simulink library "mnNb_Lib"  (R2016a)
settings: Solver=ode45  StartTime=0.0  StopTime=10.0  RelTol=1e-3
undefined symbols (not defined in the file): AA_AI, Chan, CMS_Elec, CMS_SW, FB, FB_SW, FB_SW_TTFSS, TTFSS_Elec, TTFSS_Gain
libraries: cstblocks x37, NbLibrary x33, mnNb_Lib x17
settings Model: Creator=Masayuki  LastModifiedBy=Masayuki
settings DataIOCC: LimitDataPoints=on
settings DebuggingCC: AllowSymbolicDim=off

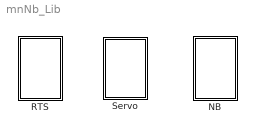
== system mnNb_Lib ==
  NB : Subsystem
  RTS : Subsystem
  Servo : Subsystem

== system mnNb_Lib/NB ==
  "NBpoint " : Subsystem  mask{DOF=''}
  NBsink : Subsystem  mask{DOF='', asd=sp}
      mask prompts: asd "Amplitude spectral density"
      mask TypeOptions asd: NbSink/asd | NbSink_CMS_CARM/asd | NbSink_CMS_IMC/asd | NbSink_FSSpath/asd | NbSink_IMCpath/asd | NbSink_TTFSS/asd | NbSink_act_AOM/asd | NbSink_act_EOM/asd | NbSink_act_IMCsus/asd | NbSink_act_PZT/asd | NbSink_act_TEMP/asd | NbSink_laser/asd | NbSink_motion_RC/asd | NbSink_seismic_CARM/asd | NbSink_seismic_IMC/asd | NbSink_shot_CARM/asd | NbSink_shot_IMC/asd | NbSink_shot_RC/asd | NbSink_sensor_IMC/asd | NbSink_sensor_RC/asd
  NoiseSource : Subsystem  mask{DOF='', group='', unit='', asd=sp}
      mask prompts: DOF "Noise name"; asd "Amplitude spectral density"
      mask TypeOptions asd: Nbsource/asd

== system mnNb_Lib/RTS ==
  ADC : Subsystem
  DAC : Subsystem
  FB_module : Subsystem
  mn Filter Bank : Subsystem  mask{Chan=Chan, FB=FB, FB_SW=FB_SW}
      mask prompts: Chan "Channel Name"; FB "FB filters container"; FB_SW "FB switch container"
      mask TypeOptions Chan: FB1/Chan | FB10/Chan | FB2/Chan | FB3/Chan | FB4/Chan | FB5/Chan | FB6/Chan | FB7/Chan | FB8/Chan | FB9/Chan
      mask TypeOptions FB: FB1/FB | FB10/FB | FB2/FB | FB3/FB | FB4/FB | FB5/FB | FB6/FB | FB7/FB | FB8/FB | FB9/FB
      mask TypeOptions FB_SW: FB1/FB_SW | FB10/FB_SW | FB2/FB_SW | FB3/FB_SW | FB4/FB_SW | FB5/FB_SW | FB6/FB_SW | FB7/FB_SW | FB8/FB_SW | FB9/FB_SW | Gain/FB_SW

== system mnNb_Lib/Servo ==
  Common Mode Servo : Subsystem  mask{CMS_Elec=CMS_Elec, CMS_SW=CMS_SW}
      mask prompts: CMS_Elec "transfer function containers"; CMS_SW "switch containers"
  TTFSS : Subsystem  mask{Elec=TTFSS_Elec, TTFSS_Gain=TTFSS_Gain, FB=FB, Chan='K1:PSL-TTFSS_TEMP_FILTER', RTS=FB_SW_TTFSS}
      mask prompts: Elec "Transfer function container"; TTFSS_Gain "Gain container"; FB "FB filters container"; Chan "Temperature control channel Name"; RTS "temperature control filters container"
      mask TypeOptions FB: TEMP Filter/FB
      mask TypeOptions Chan: TEMP Filter/Chan
      mask TypeOptions RTS: TEMP Filter/FB_SW

== system mnNb_Lib/NB/NBpoint  ==
  In1 : Inport
  NbCal : NbLibrary/NbNoiseCal  Tag=NbNoiseCal  dof=DOF  unit='control signal [V/rtHz]'
      settings: AttributesFormatString=%<Tag>
  NbSink : NbLibrary/NbNoiseSink  Tag=NbNoiseSink  dof=DOF  asd=sp  chan=''
      settings: AttributesFormatString=%<Tag>
  Sum12 : Sum  Inputs=|++
  Terminator : Terminator
  wires:
  Sum12/1 -> NbSink/1
  NbSink/1 -> Terminator/1
  In1/1 -> Sum12/1
  NbCal/1 -> Sum12/2

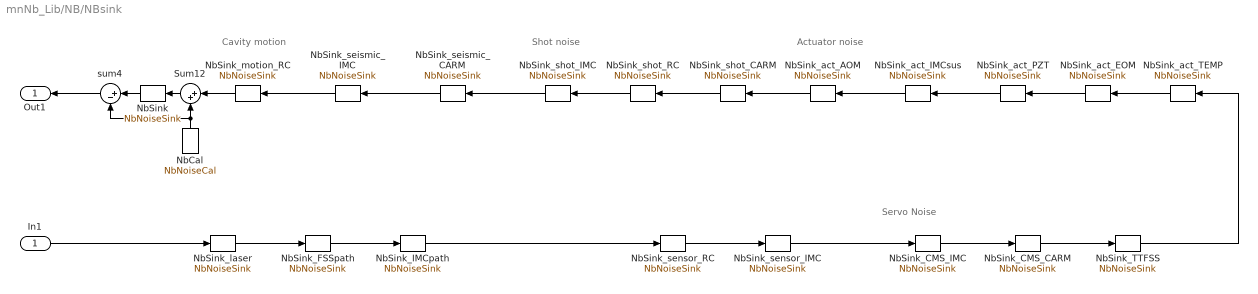
== system mnNb_Lib/NB/NBsink ==
  note: Servo Noise
  note: Actuator noise
  note: Shot noise
  note: Cavity motion
  In1 : Inport
  NbCal : NbLibrary/NbNoiseCal  Tag=NbNoiseCal  dof=DOF  unit='voltage [V/rHz]'
      settings: AttributesFormatString=%<Tag>
  NbSink : NbLibrary/NbNoiseSink  Tag=NbNoiseSink  dof=DOF  asd=sp  chan=''
      settings: AttributesFormatString=%<Tag>
  NbSink_CMS_CARM : NbLibrary/NbNoiseSink  Tag=NbNoiseSink  dof=[DOF '_CMS_CARM']  asd=sp  chan=''
      settings: AttributesFormatString=%<Tag>
  NbSink_CMS_IMC : NbLibrary/NbNoiseSink  Tag=NbNoiseSink  dof=[DOF '_CMS_IMC']  asd=sp  chan=''
      settings: AttributesFormatString=%<Tag>
  NbSink_FSSpath : NbLibrary/NbNoiseSink  Tag=NbNoiseSink  dof=[DOF '_freq_FSSpath']  asd=sp  chan=''
      settings: AttributesFormatString=%<Tag>
  NbSink_IMCpath : NbLibrary/NbNoiseSink  Tag=NbNoiseSink  dof=[DOF '_freq_IMCpath']  asd=sp  chan=''
      settings: AttributesFormatString=%<Tag>
  NbSink_TTFSS : NbLibrary/NbNoiseSink  Tag=NbNoiseSink  dof=[DOF '_TTFSS']  asd=sp  chan=''
      settings: AttributesFormatString=%<Tag>
  NbSink_act_AOM : NbLibrary/NbNoiseSink  Tag=NbNoiseSink  dof=[DOF '_act_AOM']  asd=sp  chan=''
      settings: AttributesFormatString=%<Tag>
  NbSink_act_EOM : NbLibrary/NbNoiseSink  Tag=NbNoiseSink  dof=[DOF '_act_EOM']  asd=sp  chan=''
      settings: AttributesFormatString=%<Tag>
  NbSink_act_IMCsus : NbLibrary/NbNoiseSink  Tag=NbNoiseSink  dof=[DOF '_act_IMCsus']  asd=sp  chan=''
      settings: AttributesFormatString=%<Tag>
  NbSink_act_PZT : NbLibrary/NbNoiseSink  Tag=NbNoiseSink  dof=[DOF '_act_PZT']  asd=sp  chan=''
      settings: AttributesFormatString=%<Tag>
  NbSink_act_TEMP : NbLibrary/NbNoiseSink  Tag=NbNoiseSink  dof=[DOF '_act_TEMP']  asd=sp  chan=''
      settings: AttributesFormatString=%<Tag>
  NbSink_laser : NbLibrary/NbNoiseSink  Tag=NbNoiseSink  dof=[DOF '_NPRO']  asd=sp  chan=''
      settings: AttributesFormatString=%<Tag>
  NbSink_motion_RC : NbLibrary/NbNoiseSink  Tag=NbNoiseSink  dof=[DOF '_motion_RefCav']  asd=sp  chan=''
      settings: AttributesFormatString=%<Tag>
  NbSink_seismic_CARM : NbLibrary/NbNoiseSink  Tag=NbNoiseSink  dof=[DOF '_seismic_CARM']  asd=sp  chan=''
      settings: AttributesFormatString=%<Tag>
  NbSink_seismic_IMC : NbLibrary/NbNoiseSink  Tag=NbNoiseSink  dof=[DOF '_seismic_IMC']  asd=sp  chan=''
      settings: AttributesFormatString=%<Tag>
  NbSink_sensor_IMC : NbLibrary/NbNoiseSink  Tag=NbNoiseSink  dof=[DOF '_sensor_IMC']  asd=sp  chan=''
      settings: AttributesFormatString=%<Tag>
  NbSink_sensor_RC : NbLibrary/NbNoiseSink  Tag=NbNoiseSink  dof=[DOF '_sensor_RefCav']  asd=sp  chan=''
      settings: AttributesFormatString=%<Tag>
  NbSink_shot_CARM : NbLibrary/NbNoiseSink  Tag=NbNoiseSink  dof=[DOF '_shot_CARM']  asd=sp  chan=''
      settings: AttributesFormatString=%<Tag>
  NbSink_shot_IMC : NbLibrary/NbNoiseSink  Tag=NbNoiseSink  dof=[DOF '_shot_IMC']  asd=sp  chan=''
      settings: AttributesFormatString=%<Tag>
  NbSink_shot_RC : NbLibrary/NbNoiseSink  Tag=NbNoiseSink  dof=[DOF '_shot_RefCav']  asd=sp  chan=''
      settings: AttributesFormatString=%<Tag>
  Sum12 : Sum  Inputs=|++
  sum4 : Sum  Inputs=|+-
  Out1 : Outport
  wires:
  Sum12/1 -> NbSink/1
  NbSink/1 -> sum4/1
  NbCal/1 -> sum4/2, Sum12/2
  sum4/1 -> Out1/1
  In1/1 -> NbSink_laser/1
  NbSink_motion_RC/1 -> Sum12/1
  NbSink_act_AOM/1 -> NbSink_shot_CARM/1
  NbSink_TTFSS/1 -> NbSink_act_TEMP/1
  NbSink_CMS_IMC/1 -> NbSink_CMS_CARM/1
  NbSink_shot_IMC/1 -> NbSink_seismic_CARM/1
  NbSink_shot_RC/1 -> NbSink_shot_IMC/1
  NbSink_seismic_IMC/1 -> NbSink_motion_RC/1
  NbSink_seismic_CARM/1 -> NbSink_seismic_IMC/1
  NbSink_shot_CARM/1 -> NbSink_shot_RC/1
  NbSink_act_IMCsus/1 -> NbSink_act_AOM/1
  NbSink_act_PZT/1 -> NbSink_act_IMCsus/1
  NbSink_act_EOM/1 -> NbSink_act_PZT/1
  NbSink_act_TEMP/1 -> NbSink_act_EOM/1
  NbSink_CMS_CARM/1 -> NbSink_TTFSS/1
  NbSink_laser/1 -> NbSink_FSSpath/1
  NbSink_FSSpath/1 -> NbSink_IMCpath/1
  NbSink_IMCpath/1 -> NbSink_sensor_RC/1
  NbSink_sensor_IMC/1 -> NbSink_CMS_IMC/1
  NbSink_sensor_RC/1 -> NbSink_sensor_IMC/1

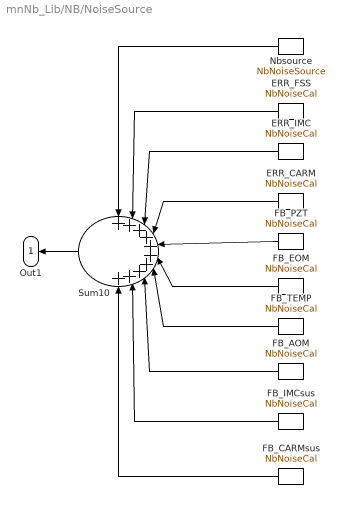
== system mnNb_Lib/NB/NoiseSource ==
  ERR_CARM : NbLibrary/NbNoiseCal  Tag=NbNoiseCal  dof=['ERR_CARM_' DOF]  unit=unit
      settings: AttributesFormatString=%<Tag>
  ERR_FSS : NbLibrary/NbNoiseCal  Tag=NbNoiseCal  dof=['ERR_FSS_' DOF]  unit=unit
      settings: AttributesFormatString=%<Tag>
  ERR_IMC : NbLibrary/NbNoiseCal  Tag=NbNoiseCal  dof=['ERR_IMC_' DOF]  unit=unit
      settings: AttributesFormatString=%<Tag>
  FB_AOM : NbLibrary/NbNoiseCal  Tag=NbNoiseCal  dof=['FB_AOM_' DOF]  unit=unit
      settings: AttributesFormatString=%<Tag>
  FB_CARMsus : NbLibrary/NbNoiseCal  Tag=NbNoiseCal  dof=['FB_CARMsus_' DOF]  unit=unit
      settings: AttributesFormatString=%<Tag>
  FB_EOM : NbLibrary/NbNoiseCal  Tag=NbNoiseCal  dof=['FB_EOM_' DOF]  unit=unit
      settings: AttributesFormatString=%<Tag>
  FB_IMCsus : NbLibrary/NbNoiseCal  Tag=NbNoiseCal  dof=['FB_IMCsus_' DOF]  unit=unit
      settings: AttributesFormatString=%<Tag>
  FB_PZT : NbLibrary/NbNoiseCal  Tag=NbNoiseCal  dof=['FB_PZT_' DOF]  unit=unit
      settings: AttributesFormatString=%<Tag>
  FB_TEMP : NbLibrary/NbNoiseCal  Tag=NbNoiseCal  dof=['FB_TEMP_' DOF]  unit=unit
      settings: AttributesFormatString=%<Tag>
  Nbsource : NbLibrary/NbNoiseSource  Tag=NbNoiseSource  asd=sp  chan=''  groupNest=1  group=group  subgroup=''  subsubgroup=''  subsubsubgroup=''
      settings: AttributesFormatString=%<Tag>
  Sum10 : Sum  Inputs=++++++++++
  Out1 : Outport
  wires:
  Nbsource/1 -> Sum10/1
  Sum10/1 -> Out1/1
  ERR_FSS/1 -> Sum10/2
  ERR_IMC/1 -> Sum10/3
  ERR_CARM/1 -> Sum10/4
  FB_PZT/1 -> Sum10/5
  FB_EOM/1 -> Sum10/6
  FB_TEMP/1 -> Sum10/7
  FB_AOM/1 -> Sum10/8
  FB_IMCsus/1 -> Sum10/9
  FB_CARMsus/1 -> Sum10/10

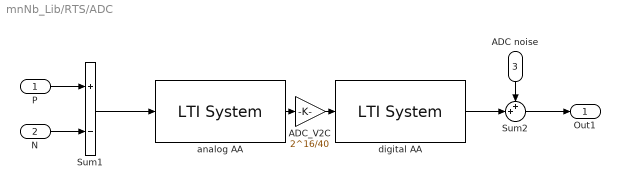
== system mnNb_Lib/RTS/ADC ==
  P : Inport
  N : Inport  Port=2
  ADC noise : Inport  Port=3
  ADC_V2C : Gain  Gain=2^16/40
  Sum1 : Sum  Inputs=+-
  Sum2 : Sum  Inputs=++|
  analog AA : cstblocks/LTI System  sys=AA_AI('Analog_AA')  IC=[]
  digital AA : cstblocks/LTI System  sys=AA_AI('Digital_AA')  IC=[]
  Out1 : Outport
  wires:
  analog AA/1 -> ADC_V2C/1
  ADC_V2C/1 -> digital AA/1
  P/1 -> Sum1/1
  N/1 -> Sum1/2
  digital AA/1 -> Sum2/2
  Sum2/1 -> Out1/1
  ADC noise/1 -> Sum2/1
  Sum1/1 -> analog AA/1

== system mnNb_Lib/RTS/DAC ==
  In1 : Inport
  DAC noise : Inport  Port=2
  DAC_C2V : Gain  Gain=20/2^16
  Sum2 : Sum  Inputs=++|
  analog AI : cstblocks/LTI System  sys=AA_AI('Analog_AI')  IC=[]
  digital AI : cstblocks/LTI System  sys=AA_AI('Digital_AI')  IC=[]
  n : Gain  Gain=-1
  P : Outport
  N : Outport  Port=2
  wires:
  In1/1 -> analog AI/1
  analog AI/1 -> DAC_C2V/1
  DAC_C2V/1 -> digital AI/1
  n/1 -> N/1
  DAC noise/1 -> Sum2/1
  digital AI/1 -> Sum2/2
  Sum2/1 -> P/1, n/1

== system mnNb_Lib/RTS/FB_module ==
  FB1 : Subsystem  mask{i=1, Chan=Chan, FB=FB, FB_SW=FB_SW}
      mask prompts: i "FB No"; Chan "Channel Name"; FB "FB filters container"; FB_SW "FB switch container"

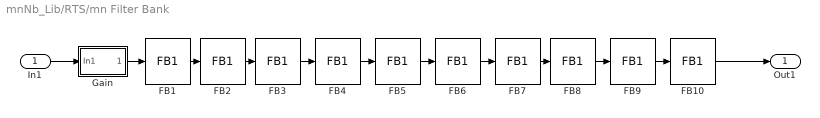
== system mnNb_Lib/RTS/mn Filter Bank ==
  In1 : Inport
  FB1 : mnNb_Lib/RTS/FB_module/FB1  i=1  Chan=Chan  FB=FB  FB_SW=FB_SW
  FB10 : mnNb_Lib/RTS/FB_module/FB1  i=10  Chan=Chan  FB=FB  FB_SW=FB_SW
  FB2 : mnNb_Lib/RTS/FB_module/FB1  i=2  Chan=Chan  FB=FB  FB_SW=FB_SW
  FB3 : mnNb_Lib/RTS/FB_module/FB1  i=3  Chan=Chan  FB=FB  FB_SW=FB_SW
  FB4 : mnNb_Lib/RTS/FB_module/FB1  i=4  Chan=Chan  FB=FB  FB_SW=FB_SW
  FB5 : mnNb_Lib/RTS/FB_module/FB1  i=5  Chan=Chan  FB=FB  FB_SW=FB_SW
  FB6 : mnNb_Lib/RTS/FB_module/FB1  i=6  Chan=Chan  FB=FB  FB_SW=FB_SW
  FB7 : mnNb_Lib/RTS/FB_module/FB1  i=7  Chan=Chan  FB=FB  FB_SW=FB_SW
  FB8 : mnNb_Lib/RTS/FB_module/FB1  i=8  Chan=Chan  FB=FB  FB_SW=FB_SW
  FB9 : mnNb_Lib/RTS/FB_module/FB1  i=9  Chan=Chan  FB=FB  FB_SW=FB_SW
  Gain : Subsystem  mask{FB_SW=FB_SW}
      mask prompts: FB_SW "gain container"
  Out1 : Outport
  wires:
  FB10/1 -> Out1/1
  FB1/1 -> FB2/1
  FB2/1 -> FB3/1
  FB3/1 -> FB4/1
  FB4/1 -> FB5/1
  FB5/1 -> FB6/1
  FB6/1 -> FB7/1
  FB7/1 -> FB8/1
  FB8/1 -> FB9/1
  FB9/1 -> FB10/1
  In1/1 -> Gain/1(In1)
  Gain/1(Out1) -> FB1/1

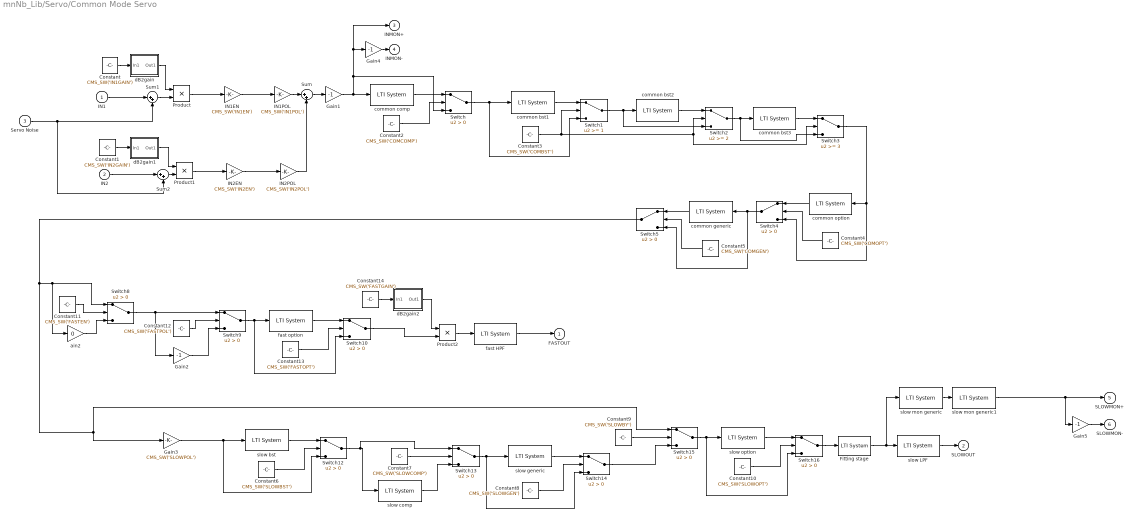
== system mnNb_Lib/Servo/Common Mode Servo ==
  IN1 : Inport
  IN2 : Inport  Port=2
  Servo Noise : Inport  Port=3
  Constant : Constant  Value=CMS_SW('IN1GAIN')
  Constant1 : Constant  Value=CMS_SW('IN2GAIN')
  Constant10 : Constant  Value=CMS_SW('SLOWOPT')
  Constant11 : Constant  Value=CMS_SW('FASTEN')
  Constant12 : Constant  Value=CMS_SW('FASTPOL')
  Constant13 : Constant  Value=CMS_SW('FASTOPT')
  Constant14 : Constant  Value=CMS_SW('FASTGAIN')
  Constant2 : Constant  Value=CMS_SW('COMCOMP')
  Constant3 : Constant  Value=CMS_SW('COMBST')
  Constant4 : Constant  Value=CMS_SW('COMOPT')
  Constant5 : Constant  Value=CMS_SW('COMGEN')
  Constant6 : Constant  Value=CMS_SW('SLOWBST')
  Constant7 : Constant  Value=CMS_SW('SLOWCOMP')
  Constant8 : Constant  Value=CMS_SW('SLOWGEN')
  Constant9 : Constant  Value=CMS_SW('SLOWBY')
  Fitting stage : cstblocks/LTI System  sys=CMS_Elec('FitStage_AOM')  IC=[]
  Gain{1..2,4..5} (4 alike) : Gain  Gain=-1
  Gain3 : Gain  Gain=CMS_SW('SLOWPOL')
  IN1EN : Gain  Gain=CMS_SW('IN1EN')
  IN1POL : Gain  Gain=CMS_SW('IN1POL')
  IN2EN : Gain  Gain=CMS_SW('IN2EN')
  IN2POL : Gain  Gain=CMS_SW('IN2POL')
  Product : Product
  Product1 : Product
  Product2 : Product
  Sum : Sum  Inputs=|++
  Sum1 : Sum  Inputs=|++
  Sum2 : Sum  Inputs=|++
  Switch{,4..5,8..10,12..16} (11 alike) : Switch  Criteria=u2 > Threshold
  Switch1 : Switch  Threshold=1
  Switch2 : Switch  Threshold=2
  Switch3 : Switch  Threshold=3
  ain2 : Gain  Gain=0
  common bst1 : cstblocks/LTI System  sys=CMS_Elec('common_bst1')  IC=[]
  common bst2 : cstblocks/LTI System  sys=CMS_Elec('common_bst2')  IC=[]
  common bst3 : cstblocks/LTI System  sys=CMS_Elec('common_bst3')  IC=[]
  common comp : cstblocks/LTI System  sys=CMS_Elec('common_comp')  IC=[]
  common generic : cstblocks/LTI System  sys=CMS_Elec('common_generic')  IC=[]
  common option : cstblocks/LTI System  sys=CMS_Elec('common_option')  IC=[]
  dB2gain : Subsystem
  dB2gain1 : Subsystem
  dB2gain2 : Subsystem
  fast HPF : cstblocks/LTI System  sys=CMS_Elec('fast_HPF')  IC=[]
  fast option : cstblocks/LTI System  sys=CMS_Elec('fast_option')  IC=[]
  slow LPF : cstblocks/LTI System  sys=CMS_Elec('slow_LPF')  IC=[]
  slow bst : cstblocks/LTI System  sys=CMS_Elec('slow_bst')  IC=[]
  slow comp : cstblocks/LTI System  sys=CMS_Elec('slow_comp')  IC=[]
  slow generic : cstblocks/LTI System  sys=CMS_Elec('slow_bst')  IC=[]
  slow mon generic : cstblocks/LTI System  sys=CMS_Elec('slow_mon_generic')  IC=[]
  slow mon generic1 : cstblocks/LTI System  sys=CMS_Elec('slow_mon_output')  IC=[]
  slow option : cstblocks/LTI System  sys=CMS_Elec('slow_option')  IC=[]
  FASTOUT : Outport
  SLOWOUT : Outport  Port=2
  INMON+ : Outport  Port=3
  INMON- : Outport  Port=4
  SLOWMON+ : Outport  Port=5
  SLOWMON- : Outport  Port=6
  wires:
  Constant/1 -> dB2gain/1(In1)
  dB2gain/1(Out1) -> Product/1
  Constant2/1 -> Switch/2
  common comp/1 -> Switch/1
  common bst1/1 -> Switch1/1
  Switch/1 -> Switch1/3, common bst1/1
  Constant3/1 -> Switch1/2, Switch2/2, Switch3/2
  Switch1/1 -> Switch2/3, common bst2/1
  common bst2/1 -> Switch2/1
  Switch2/1 -> Switch3/3, common bst3/1
  common bst3/1 -> Switch3/1
  common option/1 -> Switch4/1
  Switch3/1 -> common option/1, Switch4/3
  Constant5/1 -> Switch5/2
  common generic/1 -> Switch5/1
  Switch4/1 -> common generic/1, Switch5/3
  Constant1/1 -> dB2gain1/1(In1)
  dB2gain1/1(Out1) -> Product1/1
  Product/1 -> IN1EN/1
  IN1EN/1 -> IN1POL/1
  Product1/1 -> IN2EN/1
  IN2POL/1 -> Sum/2
  Constant6/1 -> Switch12/2
  slow bst/1 -> Switch12/1
  Gain3/1 -> slow bst/1, Switch12/3
  Constant7/1 -> Switch13/2
  Constant8/1 -> Switch14/2
  slow generic/1 -> Switch14/1
  Switch13/1 -> slow generic/1, Switch14/3
  Constant9/1 -> Switch15/2
  Switch14/1 -> Switch15/3
  Constant10/1 -> Switch16/2
  slow option/1 -> Switch16/1
  Switch15/1 -> slow option/1, Switch16/3
  slow comp/1 -> Switch13/3
  Switch12/1 -> Switch13/1, slow comp/1
  slow mon generic/1 -> slow mon generic1/1
  Gain4/1 -> INMON-/1
  Gain5/1 -> SLOWMON-/1
  Sum1/1 -> Product/2
  IN1/1 -> Sum1/1
  Sum2/1 -> Product1/2
  Servo Noise/1 -> Sum2/2, Sum1/2
  IN2/1 -> Sum2/1
  slow mon generic1/1 -> Gain5/1, SLOWMON+/1
  slow LPF/1 -> SLOWOUT/1
  Switch16/1 -> Fitting stage/1
  IN1POL/1 -> Sum/1
  IN2EN/1 -> IN2POL/1
  Constant4/1 -> Switch4/2
  Fitting stage/1 -> slow mon generic/1, slow LPF/1
  Sum/1 -> Gain1/1
  Gain1/1 -> Switch/3, INMON+/1, Gain4/1, common comp/1
  Constant11/1 -> Switch8/2
  ain2/1 -> Switch8/3
  Switch8/1 -> Switch9/1, Gain2/1
  Constant12/1 -> Switch9/2
  Gain2/1 -> Switch9/3
  Constant13/1 -> Switch10/2
  fast option/1 -> Switch10/1
  Switch9/1 -> Switch10/3, fast option/1
  Constant14/1 -> dB2gain2/1(In1)
  dB2gain2/1(Out1) -> Product2/1
  Switch10/1 -> Product2/2
  Product2/1 -> fast HPF/1
  fast HPF/1 -> FASTOUT/1
  Switch5/1 -> Gain3/1, Switch15/1, ain2/1, Switch8/1

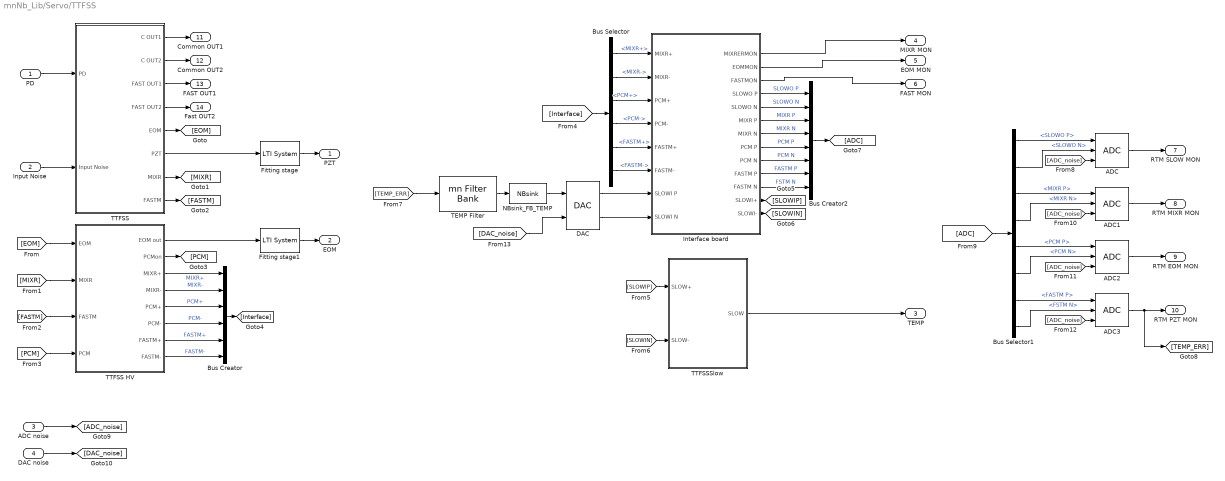
== system mnNb_Lib/Servo/TTFSS ==
  PD : Inport
  Input Noise : Inport  Port=2
  ADC noise : Inport  Port=3
  DAC noise : Inport  Port=4
  ADC{,1..3} (4 alike) : mnNb_Lib/RTS/ADC
  Bus Creator : BusCreator  Inputs=6
  Bus Creator2 : BusCreator  Inputs=8
  Bus Selector : BusSelector  OutputSignals=MIXR+,MIXR-,PCM+,PCM-,FASTM+,FASTM-
  Bus Selector1 : BusSelector  OutputSignals=SLOWO P,SLOWO N,MIXR P,MIXR N,PCM P,PCM N,FASTM P,FSTM N
  DAC : mnNb_Lib/RTS/DAC
  Fitting stage : cstblocks/LTI System  sys=Elec('FitStage_PZT')  IC=[]
  Fitting stage1 : cstblocks/LTI System  sys=Elec('FitStage_EOM')  IC=[]
  Interface board : Subsystem
  NBsink_FB_TEMP : mnNb_Lib/NB/NBsink  DOF='FB_TEMP'  asd=sp
  TEMP Filter : mnNb_Lib/RTS/mn Filter Bank  Chan=Chan  FB=FB  FB_SW=RTS
  TTFSS : Subsystem
  TTFSS HV : Subsystem
  TTFSSSlow : Subsystem
  PZT : Outport
  EOM : Outport  Port=2
  TEMP : Outport  Port=3
  MIXR MON : Outport  Port=4
  EOM MON : Outport  Port=5
  FAST MON : Outport  Port=6
  RTM SLOW MON : Outport  Port=7
  RTM MIXR MON : Outport  Port=8
  RTM EOM MON : Outport  Port=9
  RTM PZT MON : Outport  Port=10
  Common OUT1 : Outport  Port=11
  Common OUT2 : Outport  Port=12
  FAST OUT1 : Outport  Port=13
  Fast OUT2 : Outport  Port=14
  wires:
  NBsink_FB_TEMP/1 -> DAC/1
  Bus Creator2/1 -> [ADC]
  Interface board/3(FASTMON) -> FAST MON/1
  Interface board/2(EOMMON) -> EOM MON/1
  Interface board/1(MIXRERMON) -> MIXR MON/1
  [SLOWIN] -> TTFSSSlow/2(SLOW-)
  [SLOWIP] -> TTFSSSlow/1(SLOW+)
  Interface board/13(SLOWI-) -> [SLOWIN]
  Interface board/12(SLOWI+) -> [SLOWIP]
  Interface board/11(FASTM N) -> Bus Creator2/8  "FSTM N"
  Interface board/10(FASTM P) -> Bus Creator2/7  "FASTM P"
  Interface board/9(PCM N) -> Bus Creator2/6  "PCM N"
  Interface board/8(PCM P) -> Bus Creator2/5  "PCM P"
  Interface board/7(MIXR N) -> Bus Creator2/4  "MIXR N"
  Interface board/6(MIXR P) -> Bus Creator2/3  "MIXR P"
  Interface board/5(SLOWO N) -> Bus Creator2/2  "SLOWO N"
  Interface board/4(SLOWO P) -> Bus Creator2/1  "SLOWO P"
  Bus Selector/6 -> Interface board/6(FASTM-)  "<FASTM->"
  Bus Selector/4 -> Interface board/4(PCM-)  "<PCM->"
  Bus Selector/3 -> Interface board/3(PCM+)  "<PCM+>"
  Bus Selector/2 -> Interface board/2(MIXR-)  "<MIXR->"
  Bus Selector/1 -> Interface board/1(MIXR+)  "<MIXR+>"
  Bus Selector/5 -> Interface board/5(FASTM+)  "<FASTM+>"
  [Interface] -> Bus Selector/1
  Bus Creator/1 -> [Interface]
  TTFSS HV/8(FASTM-) -> Bus Creator/6  "FASTM-"
  TTFSS HV/7(FASTM+) -> Bus Creator/5  "FASTM+"
  TTFSS HV/4(MIXR-) -> Bus Creator/2  "MIXR-"
  TTFSS HV/3(MIXR+) -> Bus Creator/1  "MIXR+"
  TTFSS HV/5(PCM+) -> Bus Creator/3  "PCM+"
  TTFSS HV/6(PCM-) -> Bus Creator/4  "PCM-"
  TTFSS HV/2(PCMon) -> [PCM]
  [PCM] -> TTFSS HV/4(PCM)
  [FASTM] -> TTFSS HV/3(FASTM)
  [MIXR] -> TTFSS HV/2(MIXR)
  TTFSS/8(FASTM) -> [FASTM]
  TTFSS/7(MIXR) -> [MIXR]
  [EOM] -> TTFSS HV/1(EOM)
  TTFSS/5(EOM) -> [EOM]
  Input Noise/1 -> TTFSS/2(Input Noise)
  PD/1 -> TTFSS/1(PD)
  [ADC] -> Bus Selector1/1
  Bus Selector1/1 -> ADC/1  "<SLOWO P>"
  Bus Selector1/2 -> ADC/2  "<SLOWO N>"
  Bus Selector1/5 -> ADC2/1  "<PCM P>"
  Bus Selector1/6 -> ADC2/2  "<PCM N>"
  Bus Selector1/7 -> ADC3/1  "<FASTM P>"
  Bus Selector1/8 -> ADC3/2  "<FSTM N>"
  ADC/1 -> RTM SLOW MON/1
  ADC2/1 -> RTM EOM MON/1
  ADC3/1 -> [TEMP_ERR], RTM PZT MON/1
  DAC/2 -> Interface board/8(SLOWI N)
  DAC/1 -> Interface board/7(SLOWI P)
  [TEMP_ERR] -> TEMP Filter/1
  TEMP Filter/1 -> NBsink_FB_TEMP/1
  TTFSS/1(C OUT1) -> Common OUT1/1
  TTFSS/2(C OUT2) -> Common OUT2/1
  TTFSS/3(FAST OUT1) -> FAST OUT1/1
  TTFSS/4(FAST OUT2) -> Fast OUT2/1
  ADC noise/1 -> [ADC_noise]
  [ADC_noise] -> ADC/3
  [ADC_noise] -> ADC2/3
  [ADC_noise] -> ADC3/3
  DAC noise/1 -> [DAC_noise]
  [DAC_noise] -> DAC/2
  TTFSS/6(PZT) -> Fitting stage/1
  TTFSS HV/1(EOM out) -> Fitting stage1/1
  TTFSSSlow/1(SLOW) -> TEMP/1
  ADC1/1 -> RTM MIXR MON/1
  [ADC_noise] -> ADC1/3
  Bus Selector1/3 -> ADC1/1  "<MIXR P>"
  Bus Selector1/4 -> ADC1/2  "<MIXR N>"
  Fitting stage/1 -> PZT/1
  Fitting stage1/1 -> EOM/1

== system mnNb_Lib/RTS/FB_module/FB1 ==
  In1 : Inport
  Constant : Constant  Value=FB_SW(num2str(i))
  FB : cstblocks/LTI System  sys=FB([Chan '_FB' num2str(i)])  IC=[]
  Switch : Switch  Criteria=u2 > Threshold
  Out1 : Outport
  wires:
  FB/1 -> Switch/1
  Constant/1 -> Switch/2
  In1/1 -> FB/1, Switch/3
  Switch/1 -> Out1/1

== system mnNb_Lib/RTS/mn Filter Bank/Gain ==
  In1 : Inport
  Gain : Gain  Gain=FB_SW('Gain')
  Out1 : Outport
  wires:
  In1/1 -> Gain/1
  Gain/1 -> Out1/1

== system mnNb_Lib/Servo/Common Mode Servo/dB2gain ==
  In1 : Inport
  Gain : Gain  Gain=1/20
  Math Function : Math  Operator=10^u  SaturateOnIntegerOverflow=on
  Out1 : Outport
  wires:
  In1/1 -> Gain/1
  Math Function/1 -> Out1/1
  Gain/1 -> Math Function/1

== system mnNb_Lib/Servo/Common Mode Servo/dB2gain1 ==
  In1 : Inport
  Gain : Gain  Gain=1/20
  Math Function : Math  Operator=10^u  SaturateOnIntegerOverflow=on
  Out1 : Outport
  wires:
  In1/1 -> Gain/1
  Math Function/1 -> Out1/1
  Gain/1 -> Math Function/1

== system mnNb_Lib/Servo/Common Mode Servo/dB2gain2 ==
  In1 : Inport
  Gain : Gain  Gain=1/20
  Math Function : Math  Operator=10^u  SaturateOnIntegerOverflow=on
  Out1 : Outport
  wires:
  In1/1 -> Gain/1
  Math Function/1 -> Out1/1
  Gain/1 -> Math Function/1

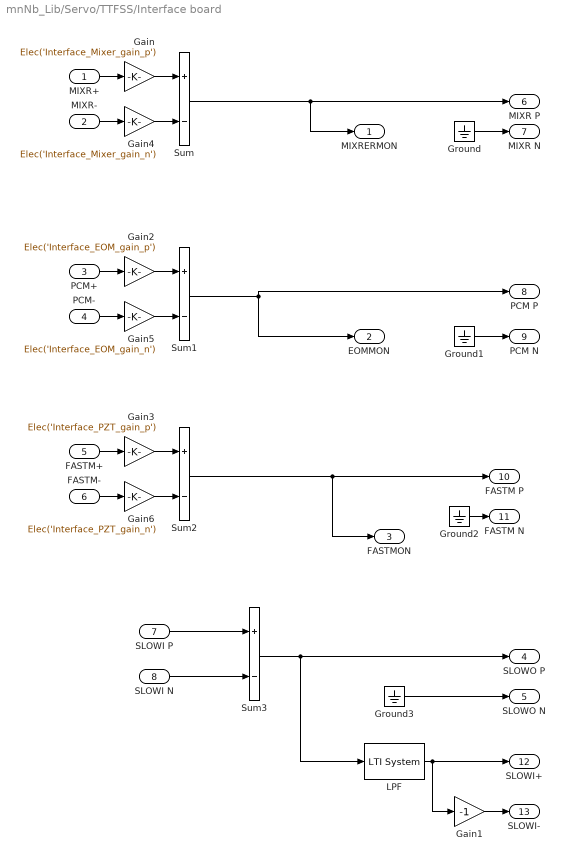
== system mnNb_Lib/Servo/TTFSS/Interface board ==
  MIXR+ : Inport
  MIXR- : Inport  Port=2
  PCM+ : Inport  Port=3
  PCM- : Inport  Port=4
  FASTM+ : Inport  Port=5
  FASTM- : Inport  Port=6
  SLOWI P : Inport  Port=7
  SLOWI N : Inport  Port=8
  Gain : Gain  Gain=Elec('Interface_Mixer_gain_p')
  Gain1 : Gain  Gain=-1
  Gain2 : Gain  Gain=Elec('Interface_EOM_gain_p')
  Gain3 : Gain  Gain=Elec('Interface_PZT_gain_p')
  Gain4 : Gain  Gain=Elec('Interface_Mixer_gain_n')
  Gain5 : Gain  Gain=Elec('Interface_EOM_gain_n')
  Gain6 : Gain  Gain=Elec('Interface_PZT_gain_n')
  Ground{,1..3} (4 alike) : Ground
  LPF : cstblocks/LTI System  sys=Elec('Interface_SLOW_LPF')  IC=[]
  Sum{,1..3} (4 alike) : Sum  Inputs=+-
  MIXRERMON : Outport
  EOMMON : Outport  Port=2
  FASTMON : Outport  Port=3
  SLOWO P : Outport  Port=4
  SLOWO N : Outport  Port=5
  MIXR P : Outport  Port=6
  MIXR N : Outport  Port=7
  PCM P : Outport  Port=8
  PCM N : Outport  Port=9
  FASTM P : Outport  Port=10
  FASTM N : Outport  Port=11
  SLOWI+ : Outport  Port=12
  SLOWI- : Outport  Port=13
  wires:
  Gain6/1 -> Sum2/2
  Gain3/1 -> Sum2/1
  FASTM+/1 -> Gain3/1
  FASTM-/1 -> Gain6/1
  Gain5/1 -> Sum1/2
  Gain2/1 -> Sum1/1
  PCM+/1 -> Gain2/1
  PCM-/1 -> Gain5/1
  Gain4/1 -> Sum/2
  Gain/1 -> Sum/1
  Gain1/1 -> SLOWI-/1
  LPF/1 -> SLOWI+/1, Gain1/1
  Ground3/1 -> SLOWO N/1
  Sum2/1 -> FASTM P/1, FASTMON/1
  Ground2/1 -> FASTM N/1
  MIXR+/1 -> Gain/1
  Sum/1 -> MIXRERMON/1, MIXR P/1
  MIXR-/1 -> Gain4/1
  Ground/1 -> MIXR N/1
  Ground1/1 -> PCM N/1
  Sum1/1 -> EOMMON/1, PCM P/1
  Sum3/1 -> LPF/1, SLOWO P/1
  SLOWI P/1 -> Sum3/1
  SLOWI N/1 -> Sum3/2

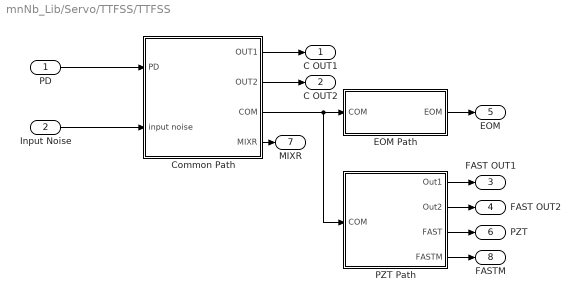
== system mnNb_Lib/Servo/TTFSS/TTFSS ==
  PD : Inport
  Input Noise : Inport  Port=2
  Common Path : Subsystem
  EOM Path : Subsystem
  PZT Path : Subsystem
  C OUT1 : Outport
  C OUT2 : Outport  Port=2
  FAST OUT1 : Outport  Port=3
  FAST OUT2 : Outport  Port=4
  EOM : Outport  Port=5
  PZT : Outport  Port=6
  MIXR : Outport  Port=7
  FASTM : Outport  Port=8
  wires:
  Common Path/4(MIXR) -> MIXR/1
  Input Noise/1 -> Common Path/2(input noise)
  PZT Path/4(FASTM) -> FASTM/1
  PZT Path/3(FAST) -> PZT/1
  PZT Path/1(Out1) -> FAST OUT1/1
  EOM Path/1(EOM) -> EOM/1
  Common Path/1(OUT1) -> C OUT1/1
  Common Path/2(OUT2) -> C OUT2/1
  PD/1 -> Common Path/1(PD)
  PZT Path/2(Out2) -> FAST OUT2/1
  Common Path/3(COM) -> PZT Path/1(COM), EOM Path/1(COM)

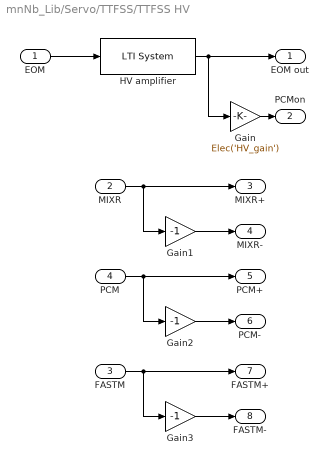
== system mnNb_Lib/Servo/TTFSS/TTFSS HV ==
  EOM : Inport
  MIXR : Inport  Port=2
  FASTM : Inport  Port=3
  PCM : Inport  Port=4
  Gain : Gain  Gain=Elec('HV_gain')
  Gain1 : Gain  Gain=-1
  Gain2 : Gain  Gain=-1
  Gain3 : Gain  Gain=-1
  HV amplifier : cstblocks/LTI System  sys=Elec('EOM_HV')  IC=[]
  EOM out : Outport
  PCMon : Outport  Port=2
  MIXR+ : Outport  Port=3
  MIXR- : Outport  Port=4
  PCM+ : Outport  Port=5
  PCM- : Outport  Port=6
  FASTM+ : Outport  Port=7
  FASTM- : Outport  Port=8
  wires:
  Gain3/1 -> FASTM-/1
  FASTM/1 -> Gain3/1, FASTM+/1
  Gain2/1 -> PCM-/1
  PCM/1 -> Gain2/1, PCM+/1
  Gain1/1 -> MIXR-/1
  MIXR/1 -> Gain1/1, MIXR+/1
  HV amplifier/1 -> EOM out/1, Gain/1
  Gain/1 -> PCMon/1
  EOM/1 -> HV amplifier/1

== system mnNb_Lib/Servo/TTFSS/TTFSSSlow ==
  SLOW+ : Inport
  SLOW- : Inport  Port=2
  SLOWn : cstblocks/LTI System  sys=Elec('SLOW_output_n')  IC=[]
  SLOWp : cstblocks/LTI System  sys=Elec('SLOW_output_p')  IC=[]
  Sum : Sum  Inputs=+-
  SLOW : Outport
  wires:
  SLOWp/1 -> Sum/1
  SLOWn/1 -> Sum/2
  SLOW-/1 -> SLOWn/1
  SLOW+/1 -> SLOWp/1
  Sum/1 -> SLOW/1

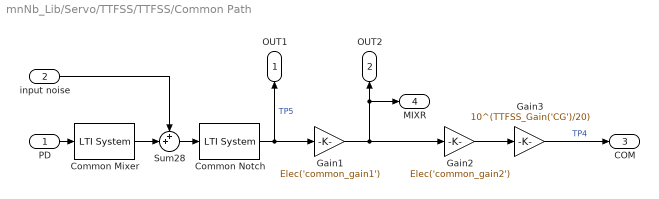
== system mnNb_Lib/Servo/TTFSS/TTFSS/Common Path ==
  PD : Inport
  input noise : Inport  Port=2
  Common Mixer : cstblocks/LTI System  sys=Elec('mixer')  IC=[]
  Common Notch : cstblocks/LTI System  sys=Elec('common_notch')  IC=[]
  Gain1 : Gain  Gain=Elec('common_gain1')
  Gain2 : Gain  Gain=Elec('common_gain2')
  Gain3 : Gain  Gain=10^(TTFSS_Gain('CG')/20)
  Sum28 : Sum  Inputs=++|
  OUT1 : Outport
  OUT2 : Outport  Port=2
  COM : Outport  Port=3
  MIXR : Outport  Port=4
  wires:
  Gain3/1 -> COM/1  "TP4"
  input noise/1 -> Sum28/1
  Sum28/1 -> Common Notch/1
  Common Mixer/1 -> Sum28/2
  Gain1/1 -> MIXR/1, OUT2/1, Gain2/1
  PD/1 -> Common Mixer/1
  Common Notch/1 -> Gain1/1, OUT1/1  "TP5"
  Gain2/1 -> Gain3/1

== system mnNb_Lib/Servo/TTFSS/TTFSS/EOM Path ==
  COM : Inport
  Add : Sum  Inputs=++|
  EOM BPF1 : cstblocks/LTI System  sys=Elec('EOM_BPF1')  IC=[]
  EOM BPF2 : cstblocks/LTI System  sys=Elec('EOM_BPF2')  IC=[]
  EOM BPF3 : cstblocks/LTI System  sys=Elec('EOM_BPF3')  IC=[]
  EOM HPF : cstblocks/LTI System  sys=Elec('EOM_HPF')  IC=[]
  EOM : Outport
  wires:
  Add/1 -> EOM/1
  EOM HPF/1 -> Add/2
  EOM BPF3/1 -> Add/1
  EOM BPF2/1 -> EOM HPF/1
  EOM BPF1/1 -> EOM BPF2/1
  COM/1 -> EOM BPF1/1, EOM BPF3/1

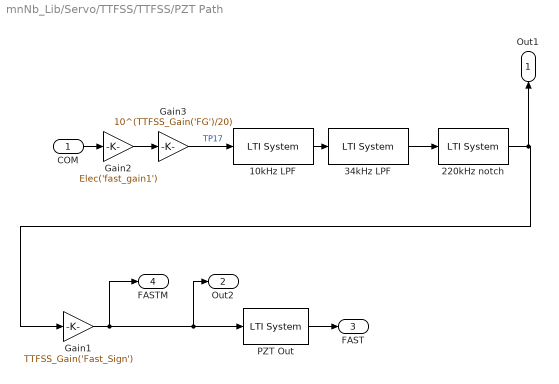
== system mnNb_Lib/Servo/TTFSS/TTFSS/PZT Path ==
  COM : Inport
  10kHz LPF : cstblocks/LTI System  sys=Elec('fast_LPF_10k')  IC=[]
  "220kHz notch " : cstblocks/LTI System  sys=Elec('fast_notch')  IC=[]
  34kHz LPF : cstblocks/LTI System  sys=Elec('fast_LPF_34k')  IC=[]
  Gain1 : Gain  Gain=TTFSS_Gain('Fast_Sign')
  Gain2 : Gain  Gain=Elec('fast_gain1')
  Gain3 : Gain  Gain=10^(TTFSS_Gain('FG')/20)
  PZT Out : cstblocks/LTI System  sys=Elec('fast_LPF_out')  IC=[]
  Out1 : Outport
  Out2 : Outport  Port=2
  FAST : Outport  Port=3
  FASTM : Outport  Port=4
  wires:
  PZT Out/1 -> FAST/1
  Gain2/1 -> Gain3/1
  10kHz LPF/1 -> 34kHz LPF/1
  COM/1 -> Gain2/1
  Gain1/1 -> Out2/1, PZT Out/1, FASTM/1
  "220kHz notch "/1 -> Out1/1, Gain1/1
  34kHz LPF/1 -> "220kHz notch "/1
  Gain3/1 -> 10kHz LPF/1  "TP17"
